simulink model "Systems_Task1_2"  (R2022a)
settings: Solver=VariableStepAuto  StartTime=0.0  StopTime=100  RelTol=1e-3
settings Model: Creator=Joel  LastModifiedBy=Joel

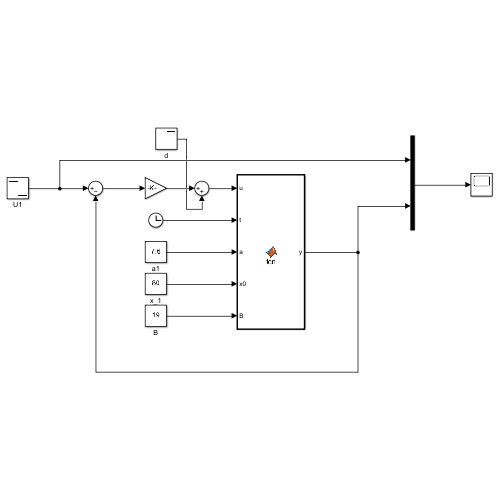
[thumbnail: Simulink's stored preview of the top-level diagram]
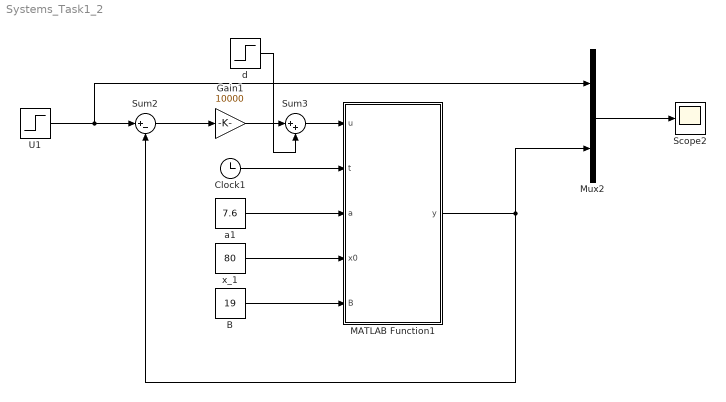
== system Systems_Task1_2 ==
  B : Constant  Value=19
  Clock1 : Clock
  Gain1 : Gain  Gain=10000
  MATLAB Function1 : MATLAB Function  TreatAsAtomicUnit=on
  Mux2 : Mux  Inputs=2
  Scope2 : Scope
  Sum2 : Sum  Inputs=|+-
  Sum3 : Sum  Inputs=|++
  U1 : Step  Time=20  Before=100  After=80  SampleTime=0
  a1 : Constant  Value=7.6
  d : Step  Time=10  After=3708  SampleTime=0
  x_1 : Constant  Value=80
  wires:
  MATLAB Function1/1(y) -> Mux2/2, Sum2/2
  x_1/1 -> MATLAB Function1/4(x0)
  a1/1 -> MATLAB Function1/3(a)
  Clock1/1 -> MATLAB Function1/2(t)
  Mux2/1 -> Scope2/1
  U1/1 -> Mux2/1, Sum2/1
  Sum2/1 -> Gain1/1
  Gain1/1 -> Sum3/1
  d/1 -> Sum3/2
  Sum3/1 -> MATLAB Function1/1(u)
  B/1 -> MATLAB Function1/5(B)

== matlab function Systems_Task1_2/MATLAB Function1 ==
  data: u input; t input; a input; x0 input; y output; B input
function y = fcn(u, t, a, x0, B)

A = x0*a -B-u;
y = (A*exp(-a*t/2560)+u+B)/a;
